simulink model "pmsm_l_portable"  (R2016a)
settings: Solver=VariableStepAuto  SolverMode=SingleTasking  StartTime=0.0  StopTime=simParam.stopTime  MaxStep=simParam.maxStep  RelTol=1e-3
values from neighbouring files (symbols this model uses):
  linear =     [linearSystem.mat]
undefined symbols (not defined in the file or in its folder): K, Ki
settings Model: Creator=KAIQUE-GCA  LastModifiedBy=kaike
settings DataIOCC: ReturnWorkspaceOutputs=on
settings DebuggingCC: UnconnectedInputMsg=none  UnconnectedOutputMsg=none  UnconnectedLineMsg=none  SFUnexpectedBacktrackingDiag=error  SFNoUnconditionalDefaultTransitionDiag=error
settings ModelReferenceCC: EnableRefExpFcnMdlSchedulingChecks=off
settings SFSimCC: SimUseLocalCustomCode=on
settings RTWCC: Description=Generic Real-Time Target  RTWUseLocalCustomCode=on
settings GRTTargetCC: TargetLangStandard=C99 (ISO)
settings ConfigComp: CovMetricSettings=dwe  CovSaveCumulativeToWorkspaceVar=off  CovSaveSingleToWorkspaceVar=off  CovExternalEMLEnable=on

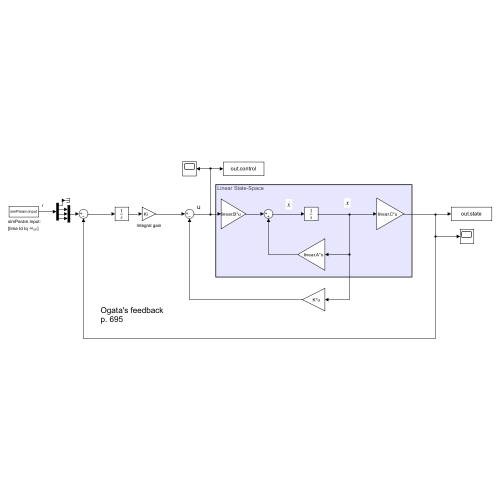
[thumbnail: Simulink's stored preview of the top-level diagram]
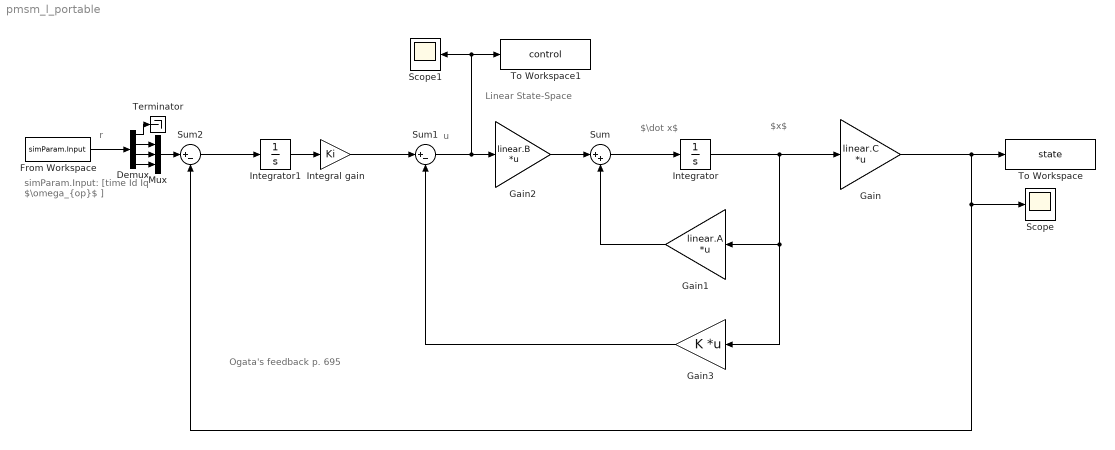
== system pmsm_l_portable ==
  note: r
  note: simParam.Input:
      | [time Id Iq $\omega_{op}$ ]
  note: u
  note: Linear State-Space
  note: Ogata's feedback
      | p. 695
  note: $x$
  note: $\dot x$
  Demux : Demux
  From Workspace : FromWorkspace  VariableName=simParam.Input  OutputAfterFinalValue=Holding final value
  Gain : Gain  Gain=linear.C  Multiplication=Matrix(K*u)
  Gain1 : Gain  Gain=linear.A  Multiplication=Matrix(K*u)
  Gain2 : Gain  Gain=linear.B  Multiplication=Matrix(K*u)
  Gain3 : Gain  Gain=K  Multiplication=Matrix(K*u)
  Integral gain : Gain  Gain=Ki
  Integrator : Integrator
  Integrator1 : Integrator
  Mux : Mux  Inputs=3
  Scope : Scope
  Scope1 : Scope
  Sum : Sum  Inputs=|++
  Sum1 : Sum  Inputs=|+-
  Sum2 : Sum  Inputs=|+-
  Terminator : Terminator
  To Workspace : ToWorkspace  VariableName=state  SampleTime=-1
  To Workspace1 : ToWorkspace  VariableName=control  SampleTime=-1
  wires:
  Sum1/1 -> Gain2/1, Scope1/1, To Workspace1/1
  Gain2/1 -> Sum/1
  Integrator/1 -> Gain3/1, Gain1/1, Gain/1
  Gain/1 -> To Workspace/1, Scope/1, Sum2/2
  Gain1/1 -> Sum/2
  Sum/1 -> Integrator/1
  Integral gain/1 -> Sum1/1
  Integrator1/1 -> Integral gain/1
  Sum2/1 -> Integrator1/1
  Gain3/1 -> Sum1/2
  Demux/2 -> Mux/1
  Demux/3 -> Mux/2
  Demux/4 -> Mux/3
  Demux/1 -> Terminator/1
  Mux/1 -> Sum2/1
  From Workspace/1 -> Demux/1
